simulink model "docking_station_model_test"  (R2023b)
settings: Solver=VariableStepDiscrete  StartTime=0.0  StopTime=86400  RelTol=1e-3
model workspace (MAT data in the model file):
  capacity = 2.7
  mean_iat = [7488 7488 7488 7488 7488 7488 936 624 468 374.4 312 267.428571429 267.428571429 267.428571429 267.428571429 234 208 187.2 208 267.428571429 374.4 468 936 3744]
  mean_iat_scalar = 2305.79761905
  n_batteries = 1
  n_docking = 3
  swap_time = 120
undefined symbols (not defined in the file or in its folder): m, n
settings Model: Creator=nimis  LastModifiedBy=nimis

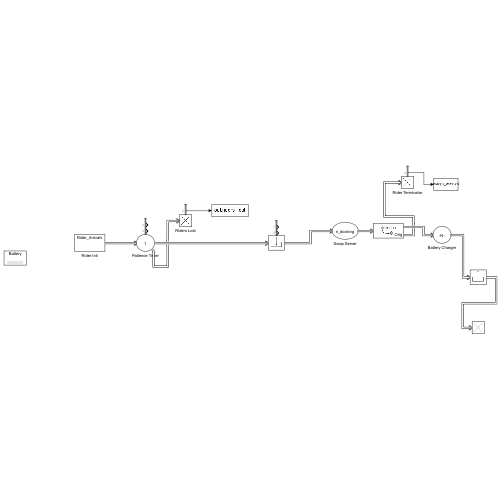
[thumbnail: Simulink's stored preview of the top-level diagram]
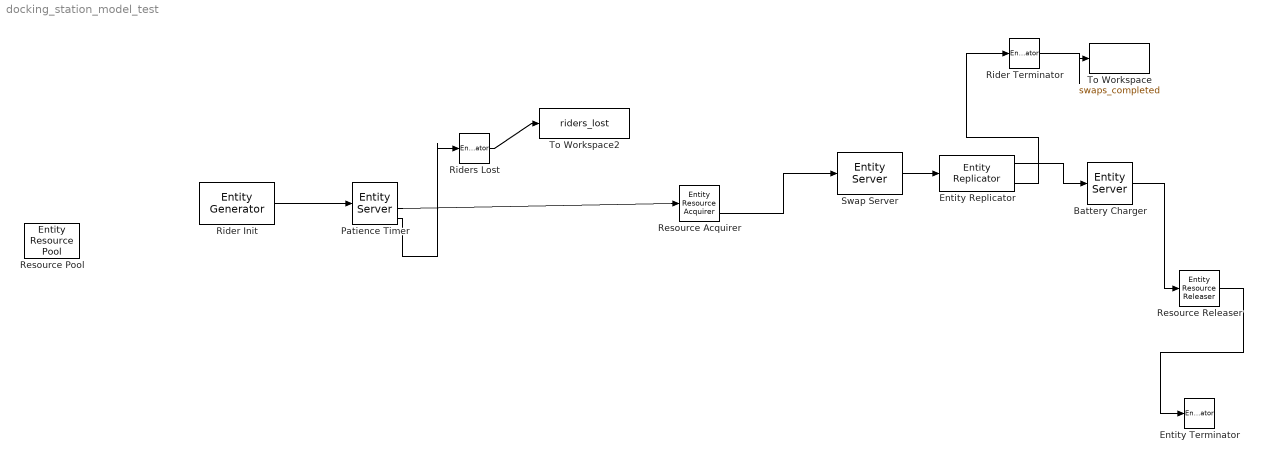
== system docking_station_model_test ==
  Battery Charger : EntityServer  InputPortMessageModes=m  OutputPortMessageModes=m  Capacity=n_docking  ServiceTimeSource=MATLAB action  ServiceTimeAction=dt = charge_time_model(entity.SOC_arrival,capacity);
  Entity Replicator : EntityReplicator  InputPortMessageModes=m  OutputPortMessageModes=m,m  ReplicasDepartFrom=Single output port
  Entity Terminator : EntityTerminator  InputPortMessageModes=m
  Patience Timer : EntityServer  InputPortMessageModes=m  OutputPortMessageModes=n,n,m,m  Capacity=1  ServiceTimeSource=Attribute  ServiceTimeAttributeName=patience  PermitPreemptionBasedOnAttribute=on  SortingAttributeName=patience  WriteResidualTimeToAttribute=on  ResidualTimeAttributeName=patience  NumberEntitiesDeparted=on  NumberEntitiesPreempted=on
      settings: OutputPortMap=o0,o6,o9,o10
  Resource Acquirer : EntityResourceAcquirer  InputPortMessageModes=m  OutputPortMessageModes=n,n,m  NumberWaitingEntities=n_docking  ResourceName=Battery  NumberEntitiesDeparted=on  NumberEntitiesInBlock=on
      settings: OutputPortMap=o0,o1,o3
  Resource Releaser : EntityResourceReleaser  InputPortMessageModes=m  OutputPortMessageModes=m
  Resource Pool : EntityResourcePool  ResourceName=Battery  ResourceAmount=n_batteries
  Rider Init : EntityGenerator  OutputPortMessageModes=m  TimeSource=MATLAB action  Period=mean_iat_scalar  IntergenerationTimeAction=|  GenerateEntityAtSimulationStart=off  AttributeName=SOC_arrival|patience  AttributeInitialValue=max(0.10, min(0.90,0.64+randn(1,1)*0.10))|300  EntityType=Structured  EntityTypeName=Rider_Arrivals
      | persistent elapsed;
      | if isempty(elapsed)
      |     elapsed = 0;
      | end
      | current_hour = floor(elapsed / 3600) + 1;
      | if current_hour > 24
      |     current_hour = 24;
      | end
      | dt = mean_iat(current_hour);
      | elapsed = elapsed + dt;
  Rider Terminator : EntityTerminator  InputPortMessageModes=m  NumberEntitiesArrived=on
      settings: OutputPortMap=o0
  Riders Lost : EntityTerminator  InputPortMessageModes=m  NumberEntitiesArrived=on
      settings: OutputPortMap=o0
  Swap Server : EntityServer  InputPortMessageModes=m  OutputPortMessageModes=m  Capacity=n_docking  ServiceTimeValue=swap_time
  To Workspace : ToWorkspace  VariableName=swaps_completed  SampleTime=-1
  To Workspace2 : ToWorkspace  VariableName=riders_lost  SampleTime=-1
  wires:
  Rider Terminator/1 -> To Workspace/1
  Swap Server/1 -> Entity Replicator/1
  Entity Replicator/2 -> Rider Terminator/1
  Entity Replicator/1 -> Battery Charger/1
  Battery Charger/1 -> Resource Releaser/1
  Resource Releaser/1 -> Entity Terminator/1
  Resource Acquirer/3 -> Swap Server/1
  Rider Init/1 -> Patience Timer/1
  Riders Lost/1 -> To Workspace2/1
  Patience Timer/3 -> Resource Acquirer/1
  Patience Timer/4 -> Riders Lost/1
